simulink model "PI_controller_windup"  (R2019b)
settings: Solver=FixedStepAuto  StartTime=0.0  StopTime=10  FixedStep=0.001  RelTol=1e-3
settings Model: Creator=suvo  LastModifiedBy=suvo

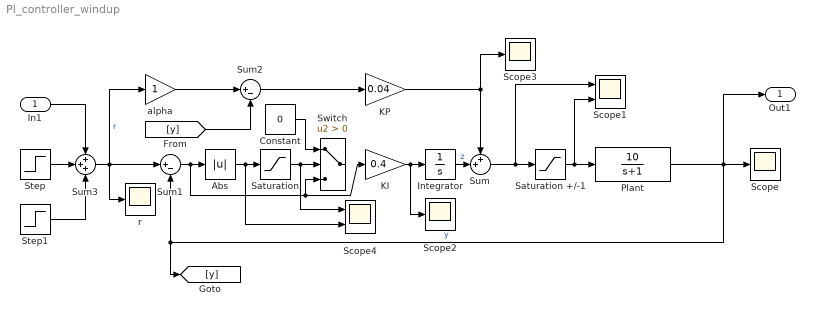
== system PI_controller_windup ==
  In1 : Inport
  Abs : Abs
  Constant : Constant  Value=0
  Integrator : Integrator
  KI : Gain  Gain=0.4
  KP : Gain  Gain=0.04
  Plant : TransferFcn  Numerator=10  Denominator=[1 1]
  Saturation : Saturate  UpperLimit=0.2  LowerLimit=-0.2
  Saturation +/-1 : Saturate  UpperLimit=0.1  LowerLimit=-0.1
  Scope : Scope
  Scope1 : Scope  NumInputPorts=2
  Scope2 : Scope
  Scope3 : Scope
  Scope4 : Scope  NumInputPorts=2
  Step : Step  Time=0  SampleTime=0
  Step1 : Step  Time=5  After=-1  SampleTime=0
  Sum : Sum  Inputs=++|
  Sum1 : Sum  Inputs=|+-
  Sum2 : Sum  Inputs=|+-
  Sum3 : Sum  Inputs=+++
  Switch : Switch  Criteria=u2 > Threshold
  alpha : Gain
  r : Scope
  Out1 : Outport
  wires:
  Plant/1 -> Scope/1, Out1/1, Sum1/2, [y]  "y"
  Sum3/1 -> r/1, alpha/1, Sum1/1  "r"
  Sum2/1 -> KP/1
  KP/1 -> Sum/1, Scope3/1
  In1/1 -> Sum3/1
  Step/1 -> Sum3/2
  [y] -> Sum2/2
  alpha/1 -> Sum2/1
  Sum/1 -> Scope1/1, Saturation +/-1/1
  Saturation +/-1/1 -> Scope1/2, Plant/1
  Step1/1 -> Sum3/3
  Integrator/1 -> Sum/2  "z"
  KI/1 -> Scope2/1, Integrator/1
  Saturation/1 -> Scope4/1, Switch/2
  Sum1/1 -> KI/1, Switch/3, Abs/1
  Abs/1 -> Scope4/2, Saturation/1
  Constant/1 -> Switch/1
